simulink library "LibEEPROM_eeprom_example_ORIGINAL"  (Simulink 10.0)
settings: Solver=VariableStepAuto  StartTime=0.0  StopTime=10.0  RelTol=1e-3
undefined symbols (not defined in the file): CRC32_calc_and_EEPROM_Write_ALL, crc32_calc_intern, CRC32_EEPROM_Read, EEPROM_Mirror, EEPROM_Read, IO_Blk_Lib_TTC500, IO_EEPROM_GetStatus, IO_EEPROM_Init, IO_EEPROM_Write, Read_Mirror, Write_Mirror, Write_Mirror_prepare_EEPROM
libraries: simulink x56
(part 2 of 8)

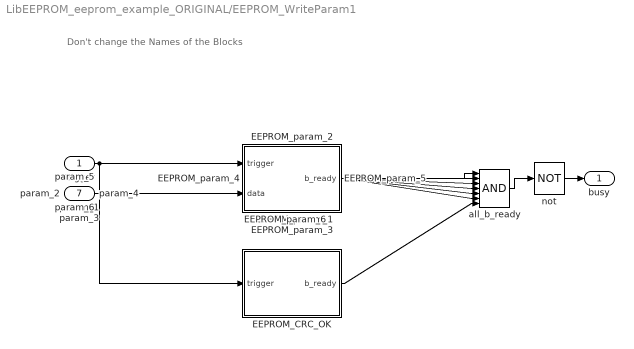
== system LibEEPROM_eeprom_example_ORIGINAL/EEPROM_WriteParam1 ==
  note: Don't change the Names of the Blocks
  trigger : Inport  OutDataTypeStr=boolean
  param_1 : Inport  Port=2
  param_2 : Inport  Port=3
  param_3 : Inport  Port=4
  param_4 : Inport  Port=5
  param_5 : Inport  Port=6
  param_6 : Inport  Port=7
  EEPROM_CRC_OK : Subsystem  LoadFcn=|  mask(CRC32_calc_and_EEPROM_Write_ALL_Code){SampleTime=-1, ttlib=IO_Blk_Lib_TTC500, ttDescription=CRC32_calc_and_EEPROM_Write_ALL, tt_iolib_version=0.16, BasicAddr=4096, EndAddr=4110, offset=4111, length=4}
      | try
      | %
      | %Upgrade Information - standard BEGIN
      | new_color = 'blue';
      | new_ver = '0.16';
      | act_ver = get_param(gcb,'tt_iolib_version');
      | if not(strcmp(act_ver,new_ver))
      |     disp(['Upgrade block: ',gcb,char(10),'       Version: ',act_ver,' -> ',new_ver]);
      |     %switch - case for specific upgrade information e.g. additional parameter required 
      |     %Change appearance and version information
      |     set_param(gcb,'ForegroundColor',new_color);
      |     set_param(gcb,'tt_iolib_version',new_ver);
      | end
      | %Upgrade Information - standard END
      | catch
      | %Standard catch section BEGIN 
      | disp(' ');
      | disp('------------------------------------------------------------');
      | disp('An error occurred in a callback of the TTC580-BlockLib.');
      | disp(['Please check the parameters in the mask of ',gcb]);
      | disp('If you do not encounter any violations, then please '); 
      | disp('copy the following lines and report this to support@ttcontrol.com ');
      | disp('<< begin of error message dump >>');
      | disp(['Version of TTC580-BlockLib: ', get_param(gcb,'tt_iolib_version')]);
      | disp(get_param(gcb,'ttDescription'));
      | disp(gcb);
      | x=lasterror;disp(x.message);
      | disp(get_param(gcb,'MaskValues'));
      | disp(version);
      | disp(computer);
      | disp('<< end of error message dump >>');
      | disp('------------------------------------------------------------');
      | disp(' ');
      | %Standard catch section END
      | end
      mask help:
      | Calculate crc32 for the section [BasicAddr .. EndAddr] out of the EEPROM and write this to a given address (=offset) in EEPROM together with all data in section [BasisAddr .. EndAddr]. This block is supposed to be used within the EEPROM_Importer() only.
      | Note: The trigger input has to be connected to the same trigger as for all EEPROM_Write blocks accessing the interval [BasicAddr .. EndAddr] otherwise data inconsitency may occur.
      mask init:
      | %
      settings: CopyFcn=%deleted
      mask Help: web(which('~.h'))
      mask Callback BasicAddr: %
      mask Callback EndAddr: %
      mask Callback offset: %
      mask Callback length: %
  EEPROM_param_1 : Subsystem  LoadFcn=|  mask(Write_Mirror_prepare_EEPROM_Code){SampleTime=-1, ttlib=IO_Blk_Lib_TTC500, ttDescription=Write_Mirror_prepare_EEPROM, tt_iolib_version=0.16, offset=4096, EEPROM_type=uint16}
      | try
      | %
      | %Upgrade Information - standard BEGIN
      | new_color = 'blue';
      | new_ver = '0.16';
      | act_ver = get_param(gcb,'tt_iolib_version');
      | if not(strcmp(act_ver,new_ver))
      |     disp(['Upgrade block: ',gcb,char(10),'       Version: ',act_ver,' -> ',new_ver]);
      |     %switch - case for specific upgrade information e.g. additional parameter required 
      |     %Change appearance and version information
      |     set_param(gcb,'ForegroundColor',new_color);
      |     set_param(gcb,'tt_iolib_version',new_ver);
      | end
      | %Upgrade Information - standard END
      | catch
      | %Standard catch section BEGIN 
      | disp(' ');
      | disp('------------------------------------------------------------');
      | disp('An error occurred in a callback of the TTC580-BlockLib.');
      | disp(['Please check the parameters in the mask of ',gcb]);
      | disp('If you do not encounter any violations, then please '); 
      | disp('copy the following lines and report this to support@ttcontrol.com ');
      | disp('<< begin of error message dump >>');
      | disp(['Version of TTC580-BlockLib: ', get_param(gcb,'tt_iolib_version')]);
      | disp(get_param(gcb,'ttDescription'));
      | disp(gcb);
      | x=lasterror;disp(x.message);
      | disp(get_param(gcb,'MaskValues'));
      | disp(version);
      | disp(computer);
      | disp('<< end of error message dump >>');
      | disp('------------------------------------------------------------');
      | disp(' ');
      | %Standard catch section END
      | end
      mask help:
      | Write data to the EEPROM_mirror[] in the context of EEPROM_Importer only.
      | Note that offset has to be in the range (0..65535).
      | Note further: No physical IO_EEPROM_Write is perfomted here. This is done in CRC32_calc_and_EEPROM_Write_ALL
      mask init:
      | try
      | switch EEPROM_type 
      |     case {'uint8'}
      |         length = 1; 
      |     case {'uint16'}; 
      |         length = 2; 
      |     case {'uint32'}
      |         length = 4; 
      |     case {'int8'}
      |         length = 1; 
      |     case {'int16'}; 
      |         length = 2; 
      |     case {'int32'}
      |         length = 4; 
      |     case {'single'}
      |         length = 4; 
      |     case {'double'}
      |         length = 8; 
      |     otherwise
      |         error('EEPROM_Write: unsupported type');
      | end
      | 
      | catch
      | %Standard catch section BEGIN 
      | disp(' ');
      | disp('------------------------------------------------------------');
      | disp('An error occurred in a callback of the TTC580-BlockLib.');
      | disp(['Please check the parameters in the mask of ',gcb]);
      | disp('If you do not encounter any violations, then please '); 
      | disp('copy the following lines and report this to support@ttcontrol.com ');
      | disp('<< begin of error message dump >>');
      | disp(['Version of TTC580-BlockLib: ', get_param(gcb,'tt_iolib_version')]);
      | disp(get_param(gcb,'ttDescription'));
      | disp(gcb);
      | x=lasterror;disp(x.message);
      | disp(get_param(gcb,'MaskValues'));
      | disp(version);
      | disp(computer);
      | disp('<< end of error message dump >>');
      | disp('------------------------------------------------------------');
      | disp(' ');
      | %Standard catch section END
      | end
      settings: CopyFcn=%deleted
      mask Help: web(which('~.h'))
      mask Callback offset: %
      mask TypeOptions EEPROM_type: uint8 | uint16 | uint32
      mask Callback EEPROM_type: %
  EEPROM_param_2 : Subsystem  LoadFcn=|  mask(Write_Mirror_prepare_EEPROM_Code){SampleTime=-1, ttlib=IO_Blk_Lib_TTC500, ttDescription=Write_Mirror_prepare_EEPROM, tt_iolib_version=0.16, offset=4098, EEPROM_type=uint16}
      | try
      | %
      | %Upgrade Information - standard BEGIN
      | new_color = 'blue';
      | new_ver = '0.16';
      | act_ver = get_param(gcb,'tt_iolib_version');
      | if not(strcmp(act_ver,new_ver))
      |     disp(['Upgrade block: ',gcb,char(10),'       Version: ',act_ver,' -> ',new_ver]);
      |     %switch - case for specific upgrade information e.g. additional parameter required 
      |     %Change appearance and version information
      |     set_param(gcb,'ForegroundColor',new_color);
      |     set_param(gcb,'tt_iolib_version',new_ver);
      | end
      | %Upgrade Information - standard END
      | catch
      | %Standard catch section BEGIN 
      | disp(' ');
      | disp('------------------------------------------------------------');
      | disp('An error occurred in a callback of the TTC580-BlockLib.');
      | disp(['Please check the parameters in the mask of ',gcb]);
      | disp('If you do not encounter any violations, then please '); 
      | disp('copy the following lines and report this to support@ttcontrol.com ');
      | disp('<< begin of error message dump >>');
      | disp(['Version of TTC580-BlockLib: ', get_param(gcb,'tt_iolib_version')]);
      | disp(get_param(gcb,'ttDescription'));
      | disp(gcb);
      | x=lasterror;disp(x.message);
      | disp(get_param(gcb,'MaskValues'));
      | disp(version);
      | disp(computer);
      | disp('<< end of error message dump >>');
      | disp('------------------------------------------------------------');
      | disp(' ');
      | %Standard catch section END
      | end
      mask help:
      | Write data to the EEPROM_mirror[] in the context of EEPROM_Importer only.
      | Note that offset has to be in the range (0..65535).
      | Note further: No physical IO_EEPROM_Write is perfomted here. This is done in CRC32_calc_and_EEPROM_Write_ALL
      mask init: same as LibEEPROM_eeprom_example_ORIGINAL/EEPROM_WriteParam1/EEPROM_param_1
      settings: CopyFcn=%deleted
      mask Help: web(which('~.h'))
      mask Callback offset: %
      mask TypeOptions EEPROM_type: uint8 | uint16 | uint32
      mask Callback EEPROM_type: %
  EEPROM_param_3 : Subsystem  LoadFcn=|  mask(Write_Mirror_prepare_EEPROM_Code){SampleTime=-1, ttlib=IO_Blk_Lib_TTC500, ttDescription=Write_Mirror_prepare_EEPROM, tt_iolib_version=0.16, offset=4100, EEPROM_type=uint8}
      | try
      | %
      | %Upgrade Information - standard BEGIN
      | new_color = 'blue';
      | new_ver = '0.16';
      | act_ver = get_param(gcb,'tt_iolib_version');
      | if not(strcmp(act_ver,new_ver))
      |     disp(['Upgrade block: ',gcb,char(10),'       Version: ',act_ver,' -> ',new_ver]);
      |     %switch - case for specific upgrade information e.g. additional parameter required 
      |     %Change appearance and version information
      |     set_param(gcb,'ForegroundColor',new_color);
      |     set_param(gcb,'tt_iolib_version',new_ver);
      | end
      | %Upgrade Information - standard END
      | catch
      | %Standard catch section BEGIN 
      | disp(' ');
      | disp('------------------------------------------------------------');
      | disp('An error occurred in a callback of the TTC580-BlockLib.');
      | disp(['Please check the parameters in the mask of ',gcb]);
      | disp('If you do not encounter any violations, then please '); 
      | disp('copy the following lines and report this to support@ttcontrol.com ');
      | disp('<< begin of error message dump >>');
      | disp(['Version of TTC580-BlockLib: ', get_param(gcb,'tt_iolib_version')]);
      | disp(get_param(gcb,'ttDescription'));
      | disp(gcb);
      | x=lasterror;disp(x.message);
      | disp(get_param(gcb,'MaskValues'));
      | disp(version);
      | disp(computer);
      | disp('<< end of error message dump >>');
      | disp('------------------------------------------------------------');
      | disp(' ');
      | %Standard catch section END
      | end
      mask help:
      | Write data to the EEPROM_mirror[] in the context of EEPROM_Importer only.
      | Note that offset has to be in the range (0..65535).
      | Note further: No physical IO_EEPROM_Write is perfomted here. This is done in CRC32_calc_and_EEPROM_Write_ALL
      mask init: same as LibEEPROM_eeprom_example_ORIGINAL/EEPROM_WriteParam1/EEPROM_param_1
      settings: CopyFcn=%deleted
      mask Help: web(which('~.h'))
      mask Callback offset: %
      mask TypeOptions EEPROM_type: uint8 | uint16 | uint32
      mask Callback EEPROM_type: %
  EEPROM_param_4 : Subsystem  LoadFcn=|  mask(Write_Mirror_prepare_EEPROM_Code){SampleTime=-1, ttlib=IO_Blk_Lib_TTC500, ttDescription=Write_Mirror_prepare_EEPROM, tt_iolib_version=0.16, offset=4101, EEPROM_type=uint32}
      | try
      | %
      | %Upgrade Information - standard BEGIN
      | new_color = 'blue';
      | new_ver = '0.16';
      | act_ver = get_param(gcb,'tt_iolib_version');
      | if not(strcmp(act_ver,new_ver))
      |     disp(['Upgrade block: ',gcb,char(10),'       Version: ',act_ver,' -> ',new_ver]);
      |     %switch - case for specific upgrade information e.g. additional parameter required 
      |     %Change appearance and version information
      |     set_param(gcb,'ForegroundColor',new_color);
      |     set_param(gcb,'tt_iolib_version',new_ver);
      | end
      | %Upgrade Information - standard END
      | catch
      | %Standard catch section BEGIN 
      | disp(' ');
      | disp('------------------------------------------------------------');
      | disp('An error occurred in a callback of the TTC580-BlockLib.');
      | disp(['Please check the parameters in the mask of ',gcb]);
      | disp('If you do not encounter any violations, then please '); 
      | disp('copy the following lines and report this to support@ttcontrol.com ');
      | disp('<< begin of error message dump >>');
      | disp(['Version of TTC580-BlockLib: ', get_param(gcb,'tt_iolib_version')]);
      | disp(get_param(gcb,'ttDescription'));
      | disp(gcb);
      | x=lasterror;disp(x.message);
      | disp(get_param(gcb,'MaskValues'));
      | disp(version);
      | disp(computer);
      | disp('<< end of error message dump >>');
      | disp('------------------------------------------------------------');
      | disp(' ');
      | %Standard catch section END
      | end
      mask help:
      | Write data to the EEPROM_mirror[] in the context of EEPROM_Importer only.
      | Note that offset has to be in the range (0..65535).
      | Note further: No physical IO_EEPROM_Write is perfomted here. This is done in CRC32_calc_and_EEPROM_Write_ALL
      mask init: same as LibEEPROM_eeprom_example_ORIGINAL/EEPROM_WriteParam1/EEPROM_param_1
      settings: CopyFcn=%deleted
      mask Help: web(which('~.h'))
      mask Callback offset: %
      mask TypeOptions EEPROM_type: uint8 | uint16 | uint32
      mask Callback EEPROM_type: %
  EEPROM_param_5 : Subsystem  LoadFcn=|  mask(Write_Mirror_prepare_EEPROM_Code){SampleTime=-1, ttlib=IO_Blk_Lib_TTC500, ttDescription=Write_Mirror_prepare_EEPROM, tt_iolib_version=0.16, offset=4105, EEPROM_type=uint32}
      | try
      | %
      | %Upgrade Information - standard BEGIN
      | new_color = 'blue';
      | new_ver = '0.16';
      | act_ver = get_param(gcb,'tt_iolib_version');
      | if not(strcmp(act_ver,new_ver))
      |     disp(['Upgrade block: ',gcb,char(10),'       Version: ',act_ver,' -> ',new_ver]);
      |     %switch - case for specific upgrade information e.g. additional parameter required 
      |     %Change appearance and version information
      |     set_param(gcb,'ForegroundColor',new_color);
      |     set_param(gcb,'tt_iolib_version',new_ver);
      | end
      | %Upgrade Information - standard END
      | catch
      | %Standard catch section BEGIN 
      | disp(' ');
      | disp('------------------------------------------------------------');
      | disp('An error occurred in a callback of the TTC580-BlockLib.');
      | disp(['Please check the parameters in the mask of ',gcb]);
      | disp('If you do not encounter any violations, then please '); 
      | disp('copy the following lines and report this to support@ttcontrol.com ');
      | disp('<< begin of error message dump >>');
      | disp(['Version of TTC580-BlockLib: ', get_param(gcb,'tt_iolib_version')]);
      | disp(get_param(gcb,'ttDescription'));
      | disp(gcb);
      | x=lasterror;disp(x.message);
      | disp(get_param(gcb,'MaskValues'));
      | disp(version);
      | disp(computer);
      | disp('<< end of error message dump >>');
      | disp('------------------------------------------------------------');
      | disp(' ');
      | %Standard catch section END
      | end
      mask help:
      | Write data to the EEPROM_mirror[] in the context of EEPROM_Importer only.
      | Note that offset has to be in the range (0..65535).
      | Note further: No physical IO_EEPROM_Write is perfomted here. This is done in CRC32_calc_and_EEPROM_Write_ALL
      mask init: same as LibEEPROM_eeprom_example_ORIGINAL/EEPROM_WriteParam1/EEPROM_param_1
      settings: CopyFcn=%deleted
      mask Help: web(which('~.h'))
      mask Callback offset: %
      mask TypeOptions EEPROM_type: uint8 | uint16 | uint32
      mask Callback EEPROM_type: %
  EEPROM_param_6 : Subsystem  LoadFcn=|  mask(Write_Mirror_prepare_EEPROM_Code){SampleTime=-1, ttlib=IO_Blk_Lib_TTC500, ttDescription=Write_Mirror_prepare_EEPROM, tt_iolib_version=0.16, offset=4109, EEPROM_type=uint16}
      | try
      | %
      | %Upgrade Information - standard BEGIN
      | new_color = 'blue';
      | new_ver = '0.16';
      | act_ver = get_param(gcb,'tt_iolib_version');
      | if not(strcmp(act_ver,new_ver))
      |     disp(['Upgrade block: ',gcb,char(10),'       Version: ',act_ver,' -> ',new_ver]);
      |     %switch - case for specific upgrade information e.g. additional parameter required 
      |     %Change appearance and version information
      |     set_param(gcb,'ForegroundColor',new_color);
      |     set_param(gcb,'tt_iolib_version',new_ver);
      | end
      | %Upgrade Information - standard END
      | catch
      | %Standard catch section BEGIN 
      | disp(' ');
      | disp('------------------------------------------------------------');
      | disp('An error occurred in a callback of the TTC580-BlockLib.');
      | disp(['Please check the parameters in the mask of ',gcb]);
      | disp('If you do not encounter any violations, then please '); 
      | disp('copy the following lines and report this to support@ttcontrol.com ');
      | disp('<< begin of error message dump >>');
      | disp(['Version of TTC580-BlockLib: ', get_param(gcb,'tt_iolib_version')]);
      | disp(get_param(gcb,'ttDescription'));
      | disp(gcb);
      | x=lasterror;disp(x.message);
      | disp(get_param(gcb,'MaskValues'));
      | disp(version);
      | disp(computer);
      | disp('<< end of error message dump >>');
      | disp('------------------------------------------------------------');
      | disp(' ');
      | %Standard catch section END
      | end
      mask help:
      | Write data to the EEPROM_mirror[] in the context of EEPROM_Importer only.
      | Note that offset has to be in the range (0..65535).
      | Note further: No physical IO_EEPROM_Write is perfomted here. This is done in CRC32_calc_and_EEPROM_Write_ALL
      mask init: same as LibEEPROM_eeprom_example_ORIGINAL/EEPROM_WriteParam1/EEPROM_param_1
      settings: CopyFcn=%deleted
      mask Help: web(which('~.h'))
      mask Callback offset: %
      mask TypeOptions EEPROM_type: uint8 | uint16 | uint32
      mask Callback EEPROM_type: %
  all_b_ready : Logic  Inputs=7  AllPortsSameDT=off  OutDataTypeStr=boolean
  not : Logic  Operator=NOT  Inputs=1  AllPortsSameDT=off  OutDataTypeStr=boolean
  busy : Outport  VectorParamsAs1DForOutWhenUnconnected=off
  wires:
  not/1 -> busy/1
  all_b_ready/1 -> not/1
  trigger/1 -> EEPROM_param_1/1(trigger), EEPROM_param_2/1(trigger), EEPROM_param_3/1(trigger), EEPROM_param_4/1(trigger), EEPROM_param_5/1(trigger), EEPROM_param_6/1(trigger), EEPROM_CRC_OK/1(trigger)
  param_1/1 -> EEPROM_param_1/2(data)
  EEPROM_param_1/1(b_ready) -> all_b_ready/1
  param_2/1 -> EEPROM_param_2/2(data)
  EEPROM_param_2/1(b_ready) -> all_b_ready/2
  param_3/1 -> EEPROM_param_3/2(data)
  EEPROM_param_3/1(b_ready) -> all_b_ready/3
  param_4/1 -> EEPROM_param_4/2(data)
  EEPROM_param_4/1(b_ready) -> all_b_ready/4
  param_5/1 -> EEPROM_param_5/2(data)
  EEPROM_param_5/1(b_ready) -> all_b_ready/5
  param_6/1 -> EEPROM_param_6/2(data)
  EEPROM_param_6/1(b_ready) -> all_b_ready/6
  EEPROM_CRC_OK/1(b_ready) -> all_b_ready/7

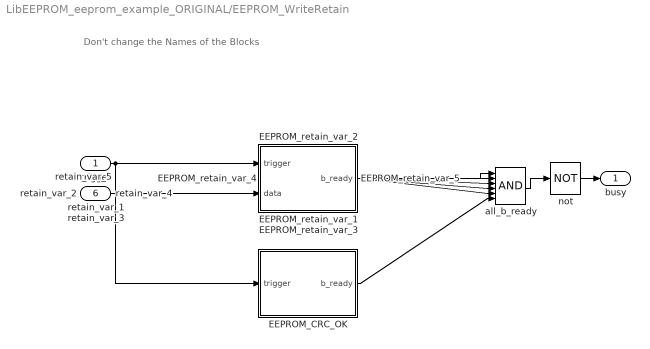
== system LibEEPROM_eeprom_example_ORIGINAL/EEPROM_WriteRetain ==
  note: Don't change the Names of the Blocks
  trigger : Inport  OutDataTypeStr=boolean
  retain_var_1 : Inport  Port=2
  retain_var_2 : Inport  Port=3
  retain_var_3 : Inport  Port=4
  retain_var_4 : Inport  Port=5
  retain_var_5 : Inport  Port=6
  EEPROM_CRC_OK : Subsystem  LoadFcn=|  mask(CRC32_calc_and_EEPROM_Write_ALL_Code){SampleTime=-1, ttlib=IO_Blk_Lib_TTC500, ttDescription=CRC32_calc_and_EEPROM_Write_ALL, tt_iolib_version=0.16, BasicAddr=8192, EndAddr=8199, offset=8200, length=4}
      | try
      | %
      | %Upgrade Information - standard BEGIN
      | new_color = 'blue';
      | new_ver = '0.16';
      | act_ver = get_param(gcb,'tt_iolib_version');
      | if not(strcmp(act_ver,new_ver))
      |     disp(['Upgrade block: ',gcb,char(10),'       Version: ',act_ver,' -> ',new_ver]);
      |     %switch - case for specific upgrade information e.g. additional parameter required 
      |     %Change appearance and version information
      |     set_param(gcb,'ForegroundColor',new_color);
      |     set_param(gcb,'tt_iolib_version',new_ver);
      | end
      | %Upgrade Information - standard END
      | catch
      | %Standard catch section BEGIN 
      | disp(' ');
      | disp('------------------------------------------------------------');
      | disp('An error occurred in a callback of the TTC580-BlockLib.');
      | disp(['Please check the parameters in the mask of ',gcb]);
      | disp('If you do not encounter any violations, then please '); 
      | disp('copy the following lines and report this to support@ttcontrol.com ');
      | disp('<< begin of error message dump >>');
      | disp(['Version of TTC580-BlockLib: ', get_param(gcb,'tt_iolib_version')]);
      | disp(get_param(gcb,'ttDescription'));
      | disp(gcb);
      | x=lasterror;disp(x.message);
      | disp(get_param(gcb,'MaskValues'));
      | disp(version);
      | disp(computer);
      | disp('<< end of error message dump >>');
      | disp('------------------------------------------------------------');
      | disp(' ');
      | %Standard catch section END
      | end
      mask help:
      | Calculate crc32 for the section [BasicAddr .. EndAddr] out of the EEPROM and write this to a given address (=offset) in EEPROM together with all data in section [BasisAddr .. EndAddr]. This block is supposed to be used within the EEPROM_Importer() only.
      | Note: The trigger input has to be connected to the same trigger as for all EEPROM_Write blocks accessing the interval [BasicAddr .. EndAddr] otherwise data inconsitency may occur.
      mask init:
      | %
      settings: CopyFcn=%deleted
      mask Help: web(which('~.h'))
      mask Callback BasicAddr: %
      mask Callback EndAddr: %
      mask Callback offset: %
      mask Callback length: %
  EEPROM_retain_var_1 : Subsystem  LoadFcn=|  mask(Write_Mirror_prepare_EEPROM_Code){SampleTime=-1, ttlib=IO_Blk_Lib_TTC500, ttDescription=Write_Mirror_prepare_EEPROM, tt_iolib_version=0.16, offset=8192, EEPROM_type=uint16}
      | try
      | %
      | %Upgrade Information - standard BEGIN
      | new_color = 'blue';
      | new_ver = '0.16';
      | act_ver = get_param(gcb,'tt_iolib_version');
      | if not(strcmp(act_ver,new_ver))
      |     disp(['Upgrade block: ',gcb,char(10),'       Version: ',act_ver,' -> ',new_ver]);
      |     %switch - case for specific upgrade information e.g. additional parameter required 
      |     %Change appearance and version information
      |     set_param(gcb,'ForegroundColor',new_color);
      |     set_param(gcb,'tt_iolib_version',new_ver);
      | end
      | %Upgrade Information - standard END
      | catch
      | %Standard catch section BEGIN 
      | disp(' ');
      | disp('------------------------------------------------------------');
      | disp('An error occurred in a callback of the TTC580-BlockLib.');
      | disp(['Please check the parameters in the mask of ',gcb]);
      | disp('If you do not encounter any violations, then please '); 
      | disp('copy the following lines and report this to support@ttcontrol.com ');
      | disp('<< begin of error message dump >>');
      | disp(['Version of TTC580-BlockLib: ', get_param(gcb,'tt_iolib_version')]);
      | disp(get_param(gcb,'ttDescription'));
      | disp(gcb);
      | x=lasterror;disp(x.message);
      | disp(get_param(gcb,'MaskValues'));
      | disp(version);
      | disp(computer);
      | disp('<< end of error message dump >>');
      | disp('------------------------------------------------------------');
      | disp(' ');
      | %Standard catch section END
      | end
      mask help:
      | Write data to the EEPROM_mirror[] in the context of EEPROM_Importer only.
      | Note that offset has to be in the range (0..65535).
      | Note further: No physical IO_EEPROM_Write is perfomted here. This is done in CRC32_calc_and_EEPROM_Write_ALL
      mask init: same as LibEEPROM_eeprom_example_ORIGINAL/EEPROM_WriteParam1/EEPROM_param_1
      settings: CopyFcn=%deleted
      mask Help: web(which('~.h'))
      mask Callback offset: %
      mask TypeOptions EEPROM_type: uint8 | uint16 | uint32
      mask Callback EEPROM_type: %
  EEPROM_retain_var_2 : Subsystem  LoadFcn=|  mask(Write_Mirror_prepare_EEPROM_Code){SampleTime=-1, ttlib=IO_Blk_Lib_TTC500, ttDescription=Write_Mirror_prepare_EEPROM, tt_iolib_version=0.16, offset=8194, EEPROM_type=uint8}
      | try
      | %
      | %Upgrade Information - standard BEGIN
      | new_color = 'blue';
      | new_ver = '0.16';
      | act_ver = get_param(gcb,'tt_iolib_version');
      | if not(strcmp(act_ver,new_ver))
      |     disp(['Upgrade block: ',gcb,char(10),'       Version: ',act_ver,' -> ',new_ver]);
      |     %switch - case for specific upgrade information e.g. additional parameter required 
      |     %Change appearance and version information
      |     set_param(gcb,'ForegroundColor',new_color);
      |     set_param(gcb,'tt_iolib_version',new_ver);
      | end
      | %Upgrade Information - standard END
      | catch
      | %Standard catch section BEGIN 
      | disp(' ');
      | disp('------------------------------------------------------------');
      | disp('An error occurred in a callback of the TTC580-BlockLib.');
      | disp(['Please check the parameters in the mask of ',gcb]);
      | disp('If you do not encounter any violations, then please '); 
      | disp('copy the following lines and report this to support@ttcontrol.com ');
      | disp('<< begin of error message dump >>');
      | disp(['Version of TTC580-BlockLib: ', get_param(gcb,'tt_iolib_version')]);
      | disp(get_param(gcb,'ttDescription'));
      | disp(gcb);
      | x=lasterror;disp(x.message);
      | disp(get_param(gcb,'MaskValues'));
      | disp(version);
      | disp(computer);
      | disp('<< end of error message dump >>');
      | disp('------------------------------------------------------------');
      | disp(' ');
      | %Standard catch section END
      | end
      mask help:
      | Write data to the EEPROM_mirror[] in the context of EEPROM_Importer only.
      | Note that offset has to be in the range (0..65535).
      | Note further: No physical IO_EEPROM_Write is perfomted here. This is done in CRC32_calc_and_EEPROM_Write_ALL
      mask init: same as LibEEPROM_eeprom_example_ORIGINAL/EEPROM_WriteParam1/EEPROM_param_1
      settings: CopyFcn=%deleted
      mask Help: web(which('~.h'))
      mask Callback offset: %
      mask TypeOptions EEPROM_type: uint8 | uint16 | uint32
      mask Callback EEPROM_type: %
  EEPROM_retain_var_3 : Subsystem  LoadFcn=|  mask(Write_Mirror_prepare_EEPROM_Code){SampleTime=-1, ttlib=IO_Blk_Lib_TTC500, ttDescription=Write_Mirror_prepare_EEPROM, tt_iolib_version=0.16, offset=8195, EEPROM_type=uint8}
      | try
      | %
      | %Upgrade Information - standard BEGIN
      | new_color = 'blue';
      | new_ver = '0.16';
      | act_ver = get_param(gcb,'tt_iolib_version');
      | if not(strcmp(act_ver,new_ver))
      |     disp(['Upgrade block: ',gcb,char(10),'       Version: ',act_ver,' -> ',new_ver]);
      |     %switch - case for specific upgrade information e.g. additional parameter required 
      |     %Change appearance and version information
      |     set_param(gcb,'ForegroundColor',new_color);
      |     set_param(gcb,'tt_iolib_version',new_ver);
      | end
      | %Upgrade Information - standard END
      | catch
      | %Standard catch section BEGIN 
      | disp(' ');
      | disp('------------------------------------------------------------');
      | disp('An error occurred in a callback of the TTC580-BlockLib.');
      | disp(['Please check the parameters in the mask of ',gcb]);
      | disp('If you do not encounter any violations, then please '); 
      | disp('copy the following lines and report this to support@ttcontrol.com ');
      | disp('<< begin of error message dump >>');
      | disp(['Version of TTC580-BlockLib: ', get_param(gcb,'tt_iolib_version')]);
      | disp(get_param(gcb,'ttDescription'));
      | disp(gcb);
      | x=lasterror;disp(x.message);
      | disp(get_param(gcb,'MaskValues'));
      | disp(version);
      | disp(computer);
      | disp('<< end of error message dump >>');
      | disp('------------------------------------------------------------');
      | disp(' ');
      | %Standard catch section END
      | end
      mask help:
      | Write data to the EEPROM_mirror[] in the context of EEPROM_Importer only.
      | Note that offset has to be in the range (0..65535).
      | Note further: No physical IO_EEPROM_Write is perfomted here. This is done in CRC32_calc_and_EEPROM_Write_ALL
      mask init: same as LibEEPROM_eeprom_example_ORIGINAL/EEPROM_WriteParam1/EEPROM_param_1
      settings: CopyFcn=%deleted
      mask Help: web(which('~.h'))
      mask Callback offset: %
      mask TypeOptions EEPROM_type: uint8 | uint16 | uint32
      mask Callback EEPROM_type: %
  EEPROM_retain_var_4 : Subsystem  LoadFcn=|  mask(Write_Mirror_prepare_EEPROM_Code){SampleTime=-1, ttlib=IO_Blk_Lib_TTC500, ttDescription=Write_Mirror_prepare_EEPROM, tt_iolib_version=0.16, offset=8196, EEPROM_type=uint16}
      | try
      | %
      | %Upgrade Information - standard BEGIN
      | new_color = 'blue';
      | new_ver = '0.16';
      | act_ver = get_param(gcb,'tt_iolib_version');
      | if not(strcmp(act_ver,new_ver))
      |     disp(['Upgrade block: ',gcb,char(10),'       Version: ',act_ver,' -> ',new_ver]);
      |     %switch - case for specific upgrade information e.g. additional parameter required 
      |     %Change appearance and version information
      |     set_param(gcb,'ForegroundColor',new_color);
      |     set_param(gcb,'tt_iolib_version',new_ver);
      | end
      | %Upgrade Information - standard END
      | catch
      | %Standard catch section BEGIN 
      | disp(' ');
      | disp('------------------------------------------------------------');
      | disp('An error occurred in a callback of the TTC580-BlockLib.');
      | disp(['Please check the parameters in the mask of ',gcb]);
      | disp('If you do not encounter any violations, then please '); 
      | disp('copy the following lines and report this to support@ttcontrol.com ');
      | disp('<< begin of error message dump >>');
      | disp(['Version of TTC580-BlockLib: ', get_param(gcb,'tt_iolib_version')]);
      | disp(get_param(gcb,'ttDescription'));
      | disp(gcb);
      | x=lasterror;disp(x.message);
      | disp(get_param(gcb,'MaskValues'));
      | disp(version);
      | disp(computer);
      | disp('<< end of error message dump >>');
      | disp('------------------------------------------------------------');
      | disp(' ');
      | %Standard catch section END
      | end
      mask help:
      | Write data to the EEPROM_mirror[] in the context of EEPROM_Importer only.
      | Note that offset has to be in the range (0..65535).
      | Note further: No physical IO_EEPROM_Write is perfomted here. This is done in CRC32_calc_and_EEPROM_Write_ALL
      mask init: same as LibEEPROM_eeprom_example_ORIGINAL/EEPROM_WriteParam1/EEPROM_param_1
      settings: CopyFcn=%deleted
      mask Help: web(which('~.h'))
      mask Callback offset: %
      mask TypeOptions EEPROM_type: uint8 | uint16 | uint32
      mask Callback EEPROM_type: %
  EEPROM_retain_var_5 : Subsystem  LoadFcn=|  mask(Write_Mirror_prepare_EEPROM_Code){SampleTime=-1, ttlib=IO_Blk_Lib_TTC500, ttDescription=Write_Mirror_prepare_EEPROM, tt_iolib_version=0.16, offset=8198, EEPROM_type=uint16}
      | try
      | %
      | %Upgrade Information - standard BEGIN
      | new_color = 'blue';
      | new_ver = '0.16';
      | act_ver = get_param(gcb,'tt_iolib_version');
      | if not(strcmp(act_ver,new_ver))
      |     disp(['Upgrade block: ',gcb,char(10),'       Version: ',act_ver,' -> ',new_ver]);
      |     %switch - case for specific upgrade information e.g. additional parameter required 
      |     %Change appearance and version information
      |     set_param(gcb,'ForegroundColor',new_color);
      |     set_param(gcb,'tt_iolib_version',new_ver);
      | end
      | %Upgrade Information - standard END
      | catch
      | %Standard catch section BEGIN 
      | disp(' ');
      | disp('------------------------------------------------------------');
      | disp('An error occurred in a callback of the TTC580-BlockLib.');
      | disp(['Please check the parameters in the mask of ',gcb]);
      | disp('If you do not encounter any violations, then please '); 
      | disp('copy the following lines and report this to support@ttcontrol.com ');
      | disp('<< begin of error message dump >>');
      | disp(['Version of TTC580-BlockLib: ', get_param(gcb,'tt_iolib_version')]);
      | disp(get_param(gcb,'ttDescription'));
      | disp(gcb);
      | x=lasterror;disp(x.message);
      | disp(get_param(gcb,'MaskValues'));
      | disp(version);
      | disp(computer);
      | disp('<< end of error message dump >>');
      | disp('------------------------------------------------------------');
      | disp(' ');
      | %Standard catch section END
      | end
      mask help:
      | Write data to the EEPROM_mirror[] in the context of EEPROM_Importer only.
      | Note that offset has to be in the range (0..65535).
      | Note further: No physical IO_EEPROM_Write is perfomted here. This is done in CRC32_calc_and_EEPROM_Write_ALL
      mask init: same as LibEEPROM_eeprom_example_ORIGINAL/EEPROM_WriteParam1/EEPROM_param_1
      settings: CopyFcn=%deleted
      mask Help: web(which('~.h'))
      mask Callback offset: %
      mask TypeOptions EEPROM_type: uint8 | uint16 | uint32
      mask Callback EEPROM_type: %
  all_b_ready : Logic  Inputs=6  AllPortsSameDT=off  OutDataTypeStr=boolean
  not : Logic  Operator=NOT  Inputs=1  AllPortsSameDT=off  OutDataTypeStr=boolean
  busy : Outport  VectorParamsAs1DForOutWhenUnconnected=off
  wires:
  not/1 -> busy/1
  all_b_ready/1 -> not/1
  trigger/1 -> EEPROM_retain_var_1/1(trigger), EEPROM_retain_var_2/1(trigger), EEPROM_retain_var_3/1(trigger), EEPROM_retain_var_4/1(trigger), EEPROM_retain_var_5/1(trigger), EEPROM_CRC_OK/1(trigger)
  retain_var_1/1 -> EEPROM_retain_var_1/2(data)
  EEPROM_retain_var_1/1(b_ready) -> all_b_ready/1
  retain_var_2/1 -> EEPROM_retain_var_2/2(data)
  EEPROM_retain_var_2/1(b_ready) -> all_b_ready/2
  retain_var_3/1 -> EEPROM_retain_var_3/2(data)
  EEPROM_retain_var_3/1(b_ready) -> all_b_ready/3
  retain_var_4/1 -> EEPROM_retain_var_4/2(data)
  EEPROM_retain_var_4/1(b_ready) -> all_b_ready/4
  retain_var_5/1 -> EEPROM_retain_var_5/2(data)
  EEPROM_retain_var_5/1(b_ready) -> all_b_ready/5
  EEPROM_CRC_OK/1(b_ready) -> all_b_ready/6

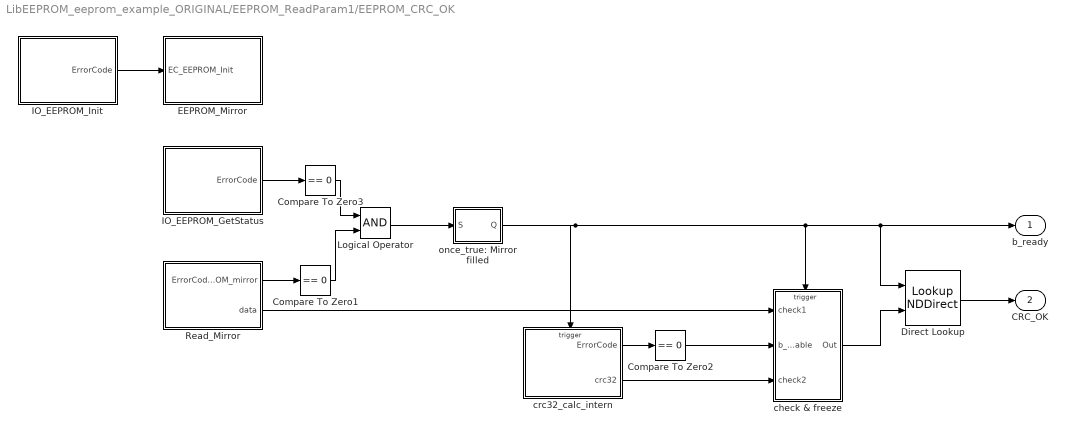
== system LibEEPROM_eeprom_example_ORIGINAL/EEPROM_ReadParam1/EEPROM_CRC_OK ==
  Compare To Zero1 : simulink/Logic and Bit Operations/Compare To Zero  relop===  OutDataTypeStr=boolean  ZeroCross=off
  Compare To Zero2 : simulink/Logic and Bit Operations/Compare To Zero  relop===  OutDataTypeStr=boolean  ZeroCross=off
  Compare To Zero3 : simulink/Logic and Bit Operations/Compare To Zero  relop===  OutDataTypeStr=boolean  ZeroCross=off
  Direct Lookup : LookupNDDirect  Table="int8([0  0;-1 1])"  DiagnosticForOutOfRangeInput=Error
  EEPROM_Mirror : Subsystem  LoadFcn=|  mask(EEPROM_Mirror_Code){SampleTime=-1, ttlib=IO_Blk_Lib_TTC500, ttDescription=EEPROM_Mirror, tt_iolib_version=0.21, offset=0, length=65536}
      | try
      | %
      | %Upgrade Information - standard BEGIN
      | new_color = 'blue';
      | new_ver = '0.21';
      | act_ver = get_param(gcb,'tt_iolib_version');
      | if not(strcmp(act_ver,new_ver))
      |     disp(['Upgrade block: ',gcb,char(10),'       Version: ',act_ver,' -> ',new_ver]);
      |     %switch - case for specific upgrade information e.g. additional parameter required 
      |     %Change appearance and version information
      |     set_param(gcb,'ForegroundColor',new_color);
      |     set_param(gcb,'tt_iolib_version',new_ver);
      | end
      | %Upgrade Information - standard END
      | catch
      | %Standard catch section BEGIN 
      | disp(' ');
      | disp('------------------------------------------------------------');
      | disp('An error occurred in a callback of the TTC580-BlockLib.');
      | disp(['Please check the parameters in the mask of ',gcb]);
      | disp('If you do not encounter any violations, then please '); 
      | disp('copy the following lines and report this to support@ttcontrol.com ');
      | disp('<< begin of error message dump >>');
      | disp(['Version of TTC580-BlockLib: ', get_param(gcb,'tt_iolib_version')]);
      | disp(get_param(gcb,'ttDescription'));
      | disp(gcb);
      | x=lasterror;disp(x.message);
      | disp(get_param(gcb,'MaskValues'));
      | disp(version);
      | disp(computer);
      | disp('<< end of error message dump >>');
      | disp('------------------------------------------------------------');
      | disp(' ');
      | %Standard catch section END
      | end
      mask help:
      | Read all data from the EEPROM and mirror this onto RAM.
      | The ErrorCode of IO_EEPROM_Init - block must be connected to the input of EEPROM_Mirror.
      | After calling EEPROM_Mirror the global variable EEPROM_mirror is filled and
      | the global variable ErrorCode_EEPROM_mirror contains the returns of IO_EEPROM_Init() and IO_EEPROM_Read().
      mask init:
      | %
      settings: CopyFcn=%deleted
      mask Help: web(which('IO_EEPROM.h'))
      mask Callback offset: %
      mask Callback length: %
  IO_EEPROM_GetStatus : Subsystem  LoadFcn=|  mask(IO_EEPROM_GetStatus_Code){SampleTime=-1, ttlib=IO_Blk_Lib_TTC500, ttDescription=IO_EEPROM_GetStatus, tt_iolib_version=0.19}
      | try
      | %
      | %Upgrade Information - standard BEGIN
      | new_color = 'blue';
      | new_ver = '0.19';
      | act_ver = get_param(gcb,'tt_iolib_version');
      | if not(strcmp(act_ver,new_ver))
      |     disp(['Upgrade block: ',gcb,char(10),'       Version: ',act_ver,' -> ',new_ver]);
      |     %switch - case for specific upgrade information e.g. additional parameter required 
      |     %Change appearance and version information
      |     set_param(gcb,'ForegroundColor',new_color);
      |     set_param(gcb,'tt_iolib_version',new_ver);
      | end
      | %Upgrade Information - standard END
      | catch
      | %Standard catch section BEGIN 
      | disp(' ');
      | disp('------------------------------------------------------------');
      | disp('An error occurred in a callback of the TTC580-BlockLib.');
      | disp(['Please check the parameters in the mask of ',gcb]);
      | disp('If you do not encounter any violations, then please '); 
      | disp('copy the following lines and report this to support@ttcontrol.com ');
      | disp('<< begin of error message dump >>');
      | disp(['Version of TTC580-BlockLib: ', get_param(gcb,'tt_iolib_version')]);
      | disp(get_param(gcb,'ttDescription'));
      | disp(gcb);
      | x=lasterror;disp(x.message);
      | disp(get_param(gcb,'MaskValues'));
      | disp(version);
      | disp(computer);
      | disp('<< end of error message dump >>');
      | disp('------------------------------------------------------------');
      | disp(' ');
      | %Standard catch section END
      | end
      mask help: Returns the status of the EEPROM driver.
      mask init:
      | %
      settings: CopyFcn=%deleted
      mask Help: web(which('IO_EEPROM.h'))
  IO_EEPROM_Init : Subsystem  LoadFcn=|  mask(IO_EEPROM_Init_Code){SampleTime=-1, ttlib=IO_Blk_Lib_TTC500, ttDescription=IO_EEPROM_Init, tt_iolib_version=0.19}
      | try
      | %
      | %Upgrade Information - standard BEGIN
      | new_color = 'blue';
      | new_ver = '0.19';
      | act_ver = get_param(gcb,'tt_iolib_version');
      | if not(strcmp(act_ver,new_ver))
      |     disp(['Upgrade block: ',gcb,char(10),'       Version: ',act_ver,' -> ',new_ver]);
      |     %switch - case for specific upgrade information e.g. additional parameter required 
      |     %Change appearance and version information
      |     set_param(gcb,'ForegroundColor',new_color);
      |     set_param(gcb,'tt_iolib_version',new_ver);
      | end
      | %Upgrade Information - standard END
      | catch
      | %Standard catch section BEGIN 
      | disp(' ');
      | disp('------------------------------------------------------------');
      | disp('An error occurred in a callback of the TTC580-BlockLib.');
      | disp(['Please check the parameters in the mask of ',gcb]);
      | disp('If you do not encounter any violations, then please '); 
      | disp('copy the following lines and report this to support@ttcontrol.com ');
      | disp('<< begin of error message dump >>');
      | disp(['Version of TTC580-BlockLib: ', get_param(gcb,'tt_iolib_version')]);
      | disp(get_param(gcb,'ttDescription'));
      | disp(gcb);
      | x=lasterror;disp(x.message);
      | disp(get_param(gcb,'MaskValues'));
      | disp(version);
      | disp(computer);
      | disp('<< end of error message dump >>');
      | disp('------------------------------------------------------------');
      | disp(' ');
      | %Standard catch section END
      | end
      mask help: Initialization of the EEPROM driver.
      mask init:
      | %
      settings: CopyFcn=%deleted
      mask Help: web(which('IO_EEPROM.h'))
  Logical Operator : Logic  AllPortsSameDT=off  OutDataTypeStr=boolean
  Read_Mirror : Subsystem  LoadFcn=|  mask(Read_Mirror_Code){SampleTime=-1, ttlib=IO_Blk_Lib_TTC500, ttDescription=Read_Mirror, tt_iolib_version=0.19, offset=offset, length=length}
      | try
      | %
      | %Upgrade Information - standard BEGIN
      | new_color = 'blue';
      | new_ver = '0.19';
      | act_ver = get_param(gcb,'tt_iolib_version');
      | if not(strcmp(act_ver,new_ver))
      |     disp(['Upgrade block: ',gcb,char(10),'       Version: ',act_ver,' -> ',new_ver]);
      |     %switch - case for specific upgrade information e.g. additional parameter required 
      |     %Change appearance and version information
      |     set_param(gcb,'ForegroundColor',new_color);
      |     set_param(gcb,'tt_iolib_version',new_ver);
      | end
      | %Upgrade Information - standard END
      | catch
      | %Standard catch section BEGIN 
      | disp(' ');
      | disp('------------------------------------------------------------');
      | disp('An error occurred in a callback of the TTC580-BlockLib.');
      | disp(['Please check the parameters in the mask of ',gcb]);
      | disp('If you do not encounter any violations, then please '); 
      | disp('copy the following lines and report this to support@ttcontrol.com ');
      | disp('<< begin of error message dump >>');
      | disp(['Version of TTC580-BlockLib: ', get_param(gcb,'tt_iolib_version')]);
      | disp(get_param(gcb,'ttDescription'));
      | disp(gcb);
      | x=lasterror;disp(x.message);
      | disp(get_param(gcb,'MaskValues'));
      | disp(version);
      | disp(computer);
      | disp('<< end of error message dump >>');
      | disp('------------------------------------------------------------');
      | disp(' ');
      | %Standard catch section END
      | end
      mask help:
      | Read data from the mirror of the EEPROM.
      | In case the given data section exceeds given EEPROM boundaries, IO_E_EEPROM_RANGE ErrorCode is returned.
      mask init:
      | %
      settings: CopyFcn=%deleted
      mask Help: web(which('~.h'))
      mask Callback offset: %
      mask Callback length: %
  check & freeze : Subsystem
  crc32_calc_intern : Subsystem  LoadFcn=|  mask(crc32_calc_intern_Code){SampleTime=-1, ttlib=IO_Blk_Lib_TTC500, ttDescription=crc32_calc_intern, tt_iolib_version=0.19, EEPROM_mirror=EEPROM_mirror, iBasicAddr_intern=BasicAddr, iEndAddr_intern=EndAddr}
      | try
      | %
      | %Upgrade Information - standard BEGIN
      | new_color = 'blue';
      | new_ver = '0.19';
      | act_ver = get_param(gcb,'tt_iolib_version');
      | if not(strcmp(act_ver,new_ver))
      |     disp(['Upgrade block: ',gcb,char(10),'       Version: ',act_ver,' -> ',new_ver]);
      |     %switch - case for specific upgrade information e.g. additional parameter required 
      |     %Change appearance and version information
      |     set_param(gcb,'ForegroundColor',new_color);
      |     set_param(gcb,'tt_iolib_version',new_ver);
      | end
      | %Upgrade Information - standard END
      | catch
      | %Standard catch section BEGIN 
      | disp(' ');
      | disp('------------------------------------------------------------');
      | disp('An error occurred in a callback of the TTC580-BlockLib.');
      | disp(['Please check the parameters in the mask of ',gcb]);
      | disp('If you do not encounter any violations, then please '); 
      | disp('copy the following lines and report this to support@ttcontrol.com ');
      | disp('<< begin of error message dump >>');
      | disp(['Version of TTC580-BlockLib: ', get_param(gcb,'tt_iolib_version')]);
      | disp(get_param(gcb,'ttDescription'));
      | disp(gcb);
      | x=lasterror;disp(x.message);
      | disp(get_param(gcb,'MaskValues'));
      | disp(version);
      | disp(computer);
      | disp('<< end of error message dump >>');
      | disp('------------------------------------------------------------');
      | disp(' ');
      | %Standard catch section END
      | end
      mask help:
      | Calculate crc32 for a section out of the EEPROM.
      | In case the given data section exceeds given EEPROM boundaries, non zero ErrorCode is returned.
      mask init:
      | %
      settings: CopyFcn=%deleted
      mask Help: No further help available for this block
      mask Callback EEPROM_mirror: %
      mask Callback iBasicAddr_intern: %
      mask Callback iEndAddr_intern: %
  once_true: Mirror filled : Subsystem  mask(SRFlipFlop){initial_condition=0}
      mask prompts: initial_condition "Initial condition (state of Q):"
      mask help: S-R Flip-Flop Block
      mask Help:
      | The S-R flip-flop also known as a set-reset flip-flop. This implementation
      | is modeled after an S-R flip-flop constructed using NOR gates. The
      | truth table for this block is:
      | <pre>
      |  S  R   Q  !Q
      |  ----------------
      |  1  0   1  0
      |  0  0   1  0  (after S == 1, R == 0)
      |  0  1   0  1
      |  0  0   0  1  (after S == 0, R == 1)
      |  1  1   0  0
      | </pre>
      | 
      | In an S-R flip-flop that is implemented with NOR gates, when a 1 is
      | applied to both the set and reset inputs, both outputs go to 0. Technically,
      | this state is undefined and is usually avoided. Note, if the flip-flop is
      | implemented with NAND gates, when a 0 is applied to both inputs, both outputs
      | go to 0 and when a 1 is applied to both inputs, the output depends on
      | the previous state of the flip-flop (previous value of Q).
  b_ready : Outport  VectorParamsAs1DForOutWhenUnconnected=off
  CRC_OK : Outport  Port=2  VectorParamsAs1DForOutWhenUnconnected=off
  wires:
  Compare To Zero2/1 -> check & freeze/2(b_enable)
  Direct Lookup/1 -> CRC_OK/1
  check & freeze/1(Out) -> Direct Lookup/2
  once_true: Mirror filled/1(Q) -> crc32_calc_intern/Trigger, check & freeze/Trigger, Direct Lookup/1, b_ready/1
  Read_Mirror/2(data) -> check & freeze/1(check1)
  crc32_calc_intern/2(crc32) -> check & freeze/3(check2)
  crc32_calc_intern/1(ErrorCode) -> Compare To Zero2/1
  Compare To Zero1/1 -> Logical Operator/2
  Compare To Zero3/1 -> Logical Operator/1
  Logical Operator/1 -> once_true: Mirror filled/1(S)
  IO_EEPROM_GetStatus/1(ErrorCode) -> Compare To Zero3/1
  IO_EEPROM_Init/1(ErrorCode) -> EEPROM_Mirror/1(EC_EEPROM_Init)
  Read_Mirror/1(ErrorCode_EEPROM_mirror) -> Compare To Zero1/1
